simulink model "Sat_Nonliner_2"  (R2024a)
settings: Solver=ode45  StartTime=0.0  StopTime=20000  RelTol=1e-3  EnableMultiTasking=on
model workspace (MAT data in the model file):
  Q_fenzi = [2.841 -4.406 1.749]
values from neighbouring files (symbols this model uses):
  sat_alpha = sat_alpha_set_3_main(sat_alpha_i)    [SAT_MAIN.m]    (also in Sat_Model_G.m = sat_alpha_set(sat_alpha_i); Sat_Model_N_P.m = sat_alpha_set(sat_alpha_i); model_sat_n_p.m = sat_alpha_1)
settings Model: Creator=75499  LastModifiedBy=xthinking
settings SolverCC: AlgebraicLoopSolver=TrustRegion
settings DataIOCC: LimitDataPoints=on  SaveFormat=Array  SignalLoggingSaveFormat=ModelDataLogs  ReturnWorkspaceOutputs=off
settings OptimizationCC: ExpressionDepthLimit=2147483647  LifeSpan=inf
settings DebuggingCC: UnderspecifiedInitializationDetection=Classic  MergeDetectMultiDrivingBlocksExec=none  SolverPrmCheckMsg=warning  FcnCallInpInsideContextMsg=warning  UnconnectedInputMsg=warning  UnconnectedOutputMsg=warning  UnconnectedLineMsg=warning  StateNameClashWarn=warning  SFUnexpectedBacktrackingDiag=warning  SFNoUnconditionalDefaultTransitionDiag=warning  SFExecutionAtInitializationDiag=none  ArithmeticOperatorsInVariantConditions=warning
settings HardwareCC: ProdBitPerPointer=32  ProdBitPerSizeT=32  ProdBitPerPtrDiffT=32  ProdLargestAtomicFloat=None  ProdIntDivRoundTo=Undefined  ProdEndianess=Unspecified  ProdWordSize=32  ProdHWDeviceType=32-bit Generic
settings ModelReferenceCC: EnableRefExpFcnMdlSchedulingChecks=on  PropagateSignalLabelsOutOfModel=off
settings SFSimCC: SimUseLocalCustomCode=off  CustomCodeUndefinedFunction=UseInterfaceOnly
settings RTWCC: RTWUseLocalCustomCode=off  GPUComputeCapability=3.5
settings CodeAppCC: StateflowObjectComments=on
settings GRTTargetCC: TargetLangStandard=C89/C90 (ANSI)
settings ConfigComp: CovMetricSettings=dw  CovSaveCumulativeToWorkspaceVar=on  CovSaveSingleToWorkspaceVar=on  CovExternalEMLEnable=off

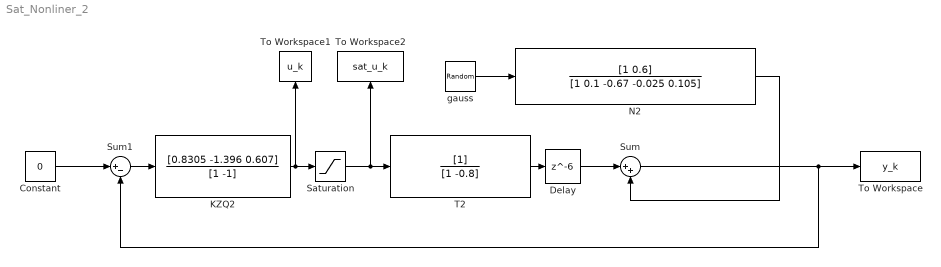
== system Sat_Nonliner_2 ==
  Constant : Constant  Value=0
  Delay : Delay  DelayLength=6
  KZQ2 : DiscreteFilter  Numerator=[0.8305 -1.396 0.607]  Denominator=[1 -1]
  N2 : DiscreteFilter  Numerator=[1 0.6]  Denominator=[1 0.1 -0.67 -0.025 0.105]
  Saturation : Saturate  UpperLimit=sat_alpha  LowerLimit=-sat_alpha  ZeroCross=off
  Sum : Sum  Inputs=|++
  Sum1 : Sum  Inputs=|+-
  T2 : DiscreteFilter  Denominator=[1 -0.8]
  To Workspace : ToWorkspace  VariableName=y_k  SampleTime=-1
  To Workspace1 : ToWorkspace  VariableName=u_k  SampleTime=-1
  To Workspace2 : ToWorkspace  VariableName=sat_u_k  SampleTime=-1
  gauss : RandomNumber  SampleTime=0.1
  wires:
  gauss/1 -> N2/1
  T2/1 -> Delay/1
  Delay/1 -> Sum/1
  N2/1 -> Sum/2
  Sum/1 -> To Workspace/1, Sum1/2
  Constant/1 -> Sum1/1
  Sum1/1 -> KZQ2/1
  Saturation/1 -> T2/1, To Workspace2/1
  KZQ2/1 -> Saturation/1, To Workspace1/1
